simulink model "SimCHinf"  (Simulink 7.5)
settings: Solver=ode45  StartTime=0.0  StopTime=100  FixedStep=0.01  MaxStep=0.01  RelTol=1e-3
values from neighbouring files (symbols this model uses):
  B = 1.1278e-3    (= 0.0011278)    [C_PID.m]
  J = 1.45e-3    (= 0.00145)    [C_PID.m]
  Ke = 0.46839    [C_PID.m]
  Kt = 0.31739    [C_PID.m]
  Ra = 6.8562    [C_PID.m]
libraries: simulink x2
settings Model: Creator=Harryth  LastModifiedBy=jorgesofrony

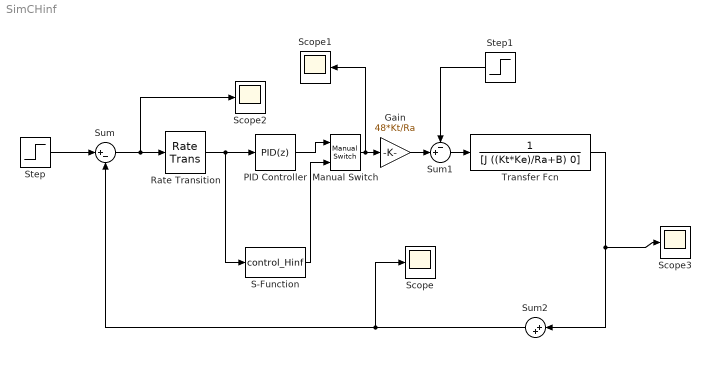
== system SimCHinf ==
  Gain : Gain  Gain=48*Kt/Ra  ParameterDataType=fixdt(1, 16)  ParameterScaling=2^0  OutDataType=fixdt(1, 16)  OutScaling=2^0
  Manual Switch : simulink/Signal Routing/Manual Switch  SystemSampleTime=-1  sw=0  action=0  varsize=off
  PID Controller : simulink/Continuous/PID Controller  DialogController=pidpack.PIDConfig.pidDDGCreate  DialogControllerArgs=DataTag0  SystemSampleTime=-1  Controller=PID  TimeDomain=Discrete-time  SampleTime=0.01  IntegratorMethod=Forward Euler  FilterMethod=Forward Euler  Form=Parallel  P=0.7  I=0.1  D=0.1  N=100  InitialConditionSource=internal  InitialConditionForIntegrator=0  InitialConditionForFilter=0  ExternalReset=none  LimitOutput=off  UpperSaturationLimit=inf  LowerSaturationLimit=-inf  LinearizeAsGain=off  AntiWindupMode=none  Kb=1  TrackingMode=off  Kt=1  PParamMin=[]  PParamMax=[]  IParamMin=[]  IParamMax=[]  DParamMin=[]  DParamMax=[]  NParamMin=[]  NParamMax=[]  KbParamMin=[]  KbParamMax=[]  KtParamMin=[]  KtParamMax=[]  POutMin=[]  POutMax=[]  IOutMin=[]  IOutMax=[]  DOutMin=[]  DOutMax=[]  NOutMin=[]  NOutMax=[]  KbOutMin=[]  KbOutMax=[]  KtOutMin=[]  KtOutMax=[]  IntegratorOutMin=[]  IntegratorOutMax=[]  FilterOutMin=[]  FilterOutMax=[]  SumOutMin=[]  SumOutMax=[]  SumI1OutMin=[]  SumI1OutMax=[]  SumI2OutMin=[]  SumI2OutMax=[]  SumI3OutMin=[]  SumI3OutMax=[]  SumDOutMin=[]  SumDOutMax=[]  SaturationOutMin=[]  SaturationOutMax=[]  IntegratorContinuousStateAttributes=''  IntegratorStateMustResolveToSignalObject=off  IntegratorRTWStateStorageClass=Auto  FilterContinuousStateAttributes=''  FilterStateMustResolveToSignalObject=off  FilterRTWStateStorageClass=Auto
  Rate Transition : RateTransition  OutPortSampleTime=0.01
  S-Function : S-Function  FunctionName=control_Hinf  Parameters=0.01  EnableBusSupport=off
  Scope{,1..3} (4 alike) : Scope
      Scope settings: YMin=5.55112e-17  YMax=1.5
      Scope1 settings: YMin=-0.12  YMax=0
      Scope2 settings: YMin=-0.1  YMax=1  SaveName=ScopeData2
      Scope3 settings: TimeRange=100  YMin=-0.3  YMax=1.4  SaveName=ScopeData3
  Step : Step  SampleTime=0
  Step1 : Step  Time=5  SampleTime=0
  Sum : Sum  Inputs=|+-
  Sum1 : Sum  Inputs=-+|
  Sum2 : Sum  Inputs=|++
  Transfer Fcn : TransferFcn  Numerator=1  Denominator=[J ((Kt*Ke)/Ra+B) 0]
  wires:
  Step/1 -> Sum/1
  Sum/1 -> Scope2/1, Rate Transition/1
  Gain/1 -> Sum1/2
  Sum1/1 -> Transfer Fcn/1
  Sum2/1 -> Sum/2, Scope/1
  Transfer Fcn/1 -> Sum2/1, Scope3/1
  Rate Transition/1 -> S-Function/1, PID Controller/1
  PID Controller/1 -> Manual Switch/1
  Manual Switch/1 -> Gain/1, Scope1/1
  S-Function/1 -> Manual Switch/2
  Step1/1 -> Sum1/1
